simulink model "FL_s_v_seno"  (R2023b)
settings: Solver=VariableStepAuto  StartTime=0.0  StopTime=50  RelTol=1e-7
settings Model: Creator=giov_russo  LastModifiedBy=miche
settings SolverCC: AlgebraicLoopSolver=TrustRegion
settings DebuggingCC: UnconnectedInputMsg=warning  UnconnectedOutputMsg=warning  UnconnectedLineMsg=warning
settings ModelReferenceCC: EnableRefExpFcnMdlSchedulingChecks=on

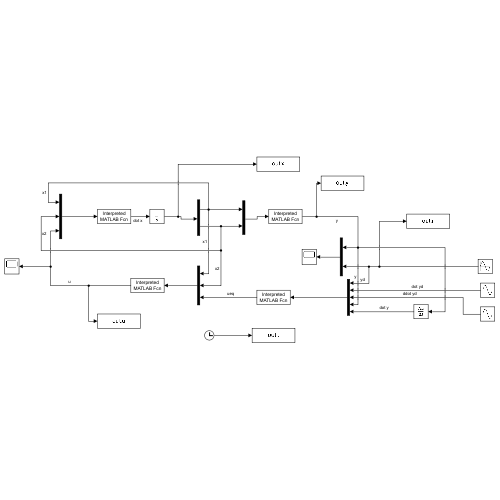
[thumbnail: Simulink's stored preview of the top-level diagram]
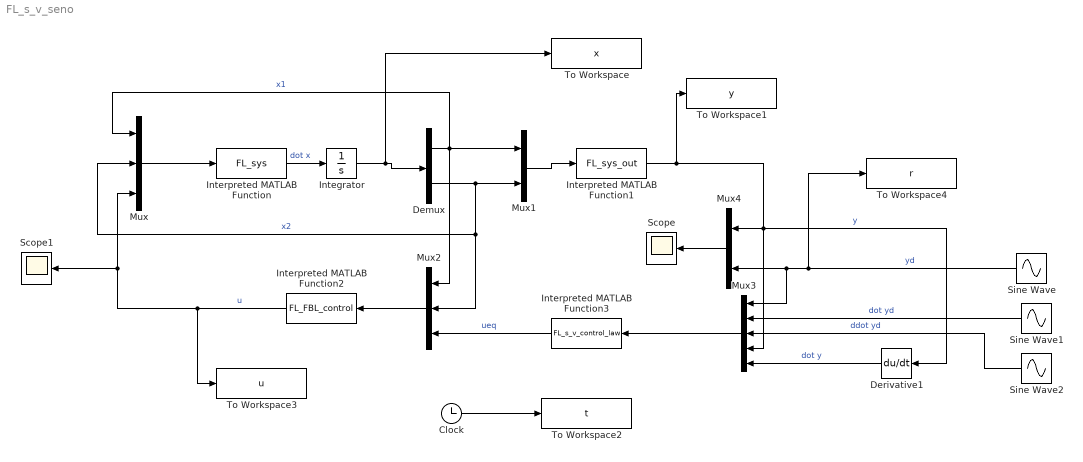
== system FL_s_v_seno ==
  Clock : Clock
  Demux : Demux  Outputs=2
  Derivative1 : Derivative
  Integrator : Integrator
  Interpreted MATLAB Function : MATLABFcn  MATLABFcn=FL_sys  OutputDimensions=2
  Interpreted MATLAB Function1 : MATLABFcn  MATLABFcn=FL_sys_out  OutputDimensions=1
  Interpreted MATLAB Function2 : MATLABFcn  MATLABFcn=FL_FBL_control  OutputDimensions=1
  Interpreted MATLAB Function3 : MATLABFcn  MATLABFcn=FL_s_v_control_law  OutputDimensions=1
  Mux : Mux  Inputs=3
  Mux1 : Mux  Inputs=2
  Mux2 : Mux  Inputs=3
  Mux3 : Mux  Inputs=5
  Mux4 : Mux  Inputs=2
  Scope : Scope
  Scope1 : Scope
  Sine Wave : Sin  Amplitude=pi  SampleTime=0
  Sine Wave1 : Sin  Amplitude=pi  Phase=pi/2  SampleTime=0
  Sine Wave2 : Sin  Amplitude=-1  SampleTime=0
  To Workspace : ToWorkspace  VariableName=x  SampleTime=-1
  To Workspace1 : ToWorkspace  VariableName=y  SampleTime=-1
  To Workspace2 : ToWorkspace  VariableName=t  SampleTime=-1
  To Workspace3 : ToWorkspace  VariableName=u  SampleTime=-1
  To Workspace4 : ToWorkspace  VariableName=r  SampleTime=-1
  wires:
  Mux/1 -> Interpreted MATLAB Function/1
  Interpreted MATLAB Function/1 -> Integrator/1  "dot x"
  Integrator/1 -> To Workspace/1, Demux/1
  Demux/2 -> Mux/2, Mux2/2, Mux1/2  "x2"
  Mux1/1 -> Interpreted MATLAB Function1/1
  Mux2/1 -> Interpreted MATLAB Function2/1
  Mux3/1 -> Interpreted MATLAB Function3/1
  Mux4/1 -> Scope/1
  Interpreted MATLAB Function2/1 -> Mux/3, Scope1/1, To Workspace3/1  "u"
  Demux/1 -> Mux/1, Mux1/1, Mux2/1  "x1"
  Interpreted MATLAB Function3/1 -> Mux2/3  "ueq"
  Interpreted MATLAB Function1/1 -> To Workspace1/1, Derivative1/1, Mux3/4, Mux4/1  "y"
  Derivative1/1 -> Mux3/5  "dot y"
  Sine Wave/1 -> To Workspace4/1, Mux3/1, Mux4/2  "yd"
  Clock/1 -> To Workspace2/1
  Sine Wave1/1 -> Mux3/2  "dot yd"
  Sine Wave2/1 -> Mux3/3  "ddot yd"
